simulink model "mbed_nucleo_f303k8_blinky"  (R2015a)
settings: Solver=FixedStepDiscrete  SolverMode=SingleTasking  StartTime=0.0  StopTime=10.0  FixedStep=1e-3  RelTol=1e-3
libraries: mbed_lib x2, mbed_targets_stm_nucleo_f303k8 x2
settings Model: CovSFcnEnable=off  Creator=oh  LastModifiedBy=oh
settings OptimizationCC: OptimizeModelRefInitCode=on  LifeSpan=1
settings DebuggingCC: SolverPrmCheckMsg=warning
settings HardwareCC: ProdLargestAtomicInteger=Long  ProdLargestAtomicFloat=Double  ProdEndianess=LittleEndian  ProdHWDeviceType=ARM Compatible->ARM Cortex
settings RTWCC: SystemTargetFile=mbed.tlc  TemplateMakefile=mbed.tmf  Description=Mbed Target (Embedded Target)  TargetLang=C++
settings CodeAppCC: IgnoreCustomStorageClasses=off
settings STFCustomTargetCC: CombineOutputUpdateFcns=on  SupportContinuousTime=off  SupportVariableSizeSignals=off  SystemTargetFile=mbed.tlc
settings ERTTargetCC: SupportContinuousTime=off  SupportVariableSizeSignals=off  ERTCustomFileTemplate=mbed_file_process.tlc

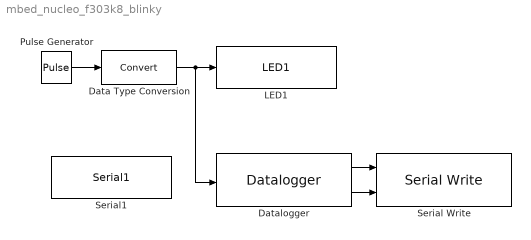
== system mbed_nucleo_f303k8_blinky ==
  Data Type Conversion : DataTypeConversion
  Datalogger : mbed_lib/Utilities/Datalogger  TypeInputPorts={ 'uint8' 1 }  TypeOfInputs={'1*uint8'}  BufferSize=100  errEn=off  SampleTime=-1
  LED1 : mbed_targets_stm_nucleo_f303k8/LED1  Parameter1=0
  Pulse Generator : DiscretePulseGenerator  PulseType=Time based  Period=1  PulseWidth=50
  Serial Write : mbed_lib/Serial/Serial Write  SerialPort=1  numData=on  SampleTime=-1
  Serial1 : mbed_targets_stm_nucleo_f303k8/Serial1  Parameter1=0  BaudRate=9600
  wires:
  Pulse Generator/1 -> Data Type Conversion/1
  Data Type Conversion/1 -> Datalogger/1, LED1/1
  Datalogger/1 -> Serial Write/1
  Datalogger/2 -> Serial Write/2
